simulink model "SwarmOptimizer"  (R2020a)
settings: Solver=VariableStepAuto  StartTime=0.0  StopTime=10.0  RelTol=1e-3
settings Model: Creator=PIM  LastModifiedBy=PIM

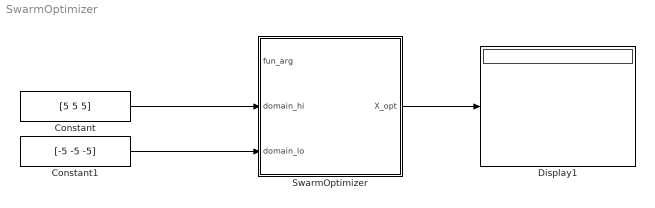
== system SwarmOptimizer ==
  Constant : Constant  Value=[5 5 5]  VectorParams1D=off
  Constant1 : Constant  Value=[-5 -5 -5]  VectorParams1D=off
  Display1 : Display
  SwarmOptimizer : Subsystem  mask{algorithm_mask=Differential Evolution Optimizer, n_iter=100, n_particles=50, sampling_method_mask=Uniform, dynamic_domain_flag=on, domain_hi_mask=[0 0 0], domain_lo_mask=[0 0 0]}
      mask prompts: algorithm_mask "Algorithm"; n_iter "Number of iterations [float]"; n_particles "Number of particles [float]"; sampling_method_mask "Sampling method"; dynamic_domain_flag "Dymamic Domain"; domain_hi_mask "Domain Hi (array) [float]"; domain_lo_mask "Domain Lo (array) [float]"
      mask init:
      | if strcmp(sampling_method_mask, 'Uniform')
      |     sampling_method=1;
      | elseif strcmp(sampling_method_mask, 'Cauchy')
      |     sampling_method=2;
      | elseif strcmp(sampling_method_mask, 'Normal')
      |     sampling_method=3;
      | end
      | 
      | if strcmp(algorithm_mask, 'Particle Swarm Optimizer')
      |     algorithm=1;
      | elseif strcmp(algorithm_mask, 'Differential Evolution Optimizer')
      |     algorithm=2;
      | end
      mask TypeOptions algorithm_mask: Particle Swarm Optimizer | Differential Evolution Optimizer
      mask TypeOptions sampling_method_mask: Uniform | Normal  | Cauchy
      mask DialogControl DescTextVar Prompt: Block to optimize a function using Swarm/Population based algorithms.
      mask DialogControl DescTextVar_copy Prompt: The function to be optimized is fun_opt(x, args)
      mask DialogControl DescTextVar_copy_copy Prompt: x: optimization variables (inputs)
      mask DialogControl DescTextVar_copy_copy_copy Prompt: args: disturbances
      mask DialogControl Control5 Prompt: Static Domain Definition
      mask Display: image('$imagefile'); % Use "Edit Image" on toolstrip to change.
  wires:
  SwarmOptimizer/1(X_opt) -> Display1/1
  Constant1/1 -> SwarmOptimizer/3(domain_lo)
  Constant/1 -> SwarmOptimizer/2(domain_hi)

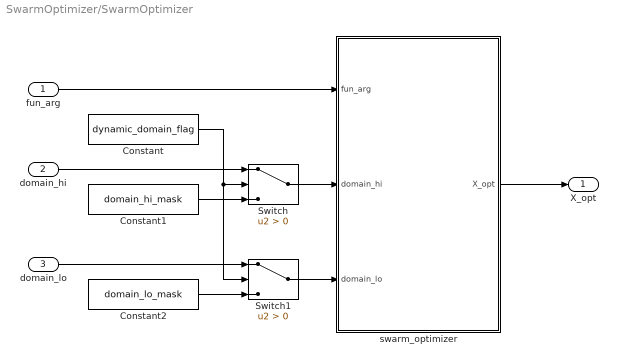
== system SwarmOptimizer/SwarmOptimizer ==
  fun_arg : Inport
  domain_hi : Inport  Port=2
  domain_lo : Inport  Port=3
  Constant : Constant  Value=dynamic_domain_flag
  Constant1 : Constant  Value=domain_hi_mask  VectorParams1D=off
  Constant2 : Constant  Value=domain_lo_mask  VectorParams1D=off
  Switch : Switch  Criteria=u2 > Threshold
  Switch1 : Switch  Criteria=u2 > Threshold
  swarm_optimizer : MATLAB Function  TreatAsAtomicUnit=on
  X_opt : Outport
  wires:
  domain_lo/1 -> Switch1/1
  Switch/1 -> swarm_optimizer/2(domain_hi)
  Constant2/1 -> Switch1/3
  Constant1/1 -> Switch/3
  Constant/1 -> Switch1/2, Switch/2
  domain_hi/1 -> Switch/1
  fun_arg/1 -> swarm_optimizer/1(fun_arg)
  Switch1/1 -> swarm_optimizer/3(domain_lo)
  swarm_optimizer/1(X_opt) -> X_opt/1

== matlab function SwarmOptimizer/swarm_optimizer ==
  data: fun_arg input; n_particles parameter int32; n_iter parameter int32; sampling_method parameter int8; algorithm parameter int8; X_opt output; domain_hi input double; domain_lo input double
function X_opt = swarm_optimizer(fun_arg, n_particles, n_iter, sampling_method, algorithm, domain_hi, domain_lo)
% global swarm_obj
% global topology_obj

swarm_obj=swarm;
topology_obj=topology;

%% Swarm parameters
swarm_param.n_particles=n_particles;
swarm_param.sampling_method='Uniform';
if sampling_method==1
    swarm_param.sampling_method='Uniform';
elseif sampling_method==2
    swarm_param.sampling_method='Cauchy';
elseif sampling_method==3
    swarm_param.sampling_method='Normal';
end
swarm_param.x_domain.hi=domain_hi;
swarm_param.x_domain.lo=domain_lo;

%% Algorithm parameters
alg_param.n_iter=n_iter;

alg_param.algorithm='ParticleSwarmOptimizer';
if algorithm==1
    alg_param.algorithm='ParticleSwarmOptimizer';
elseif algorithm==2
    alg_param.algorithm='DifferentialEvolutionOptimizer';
end


%% Specific configurations for Differential Evolution Algorithm
alg_param.CR    =0.9;       % crossover probability [0, 1]
alg_param.F     =0.8;       % differential weight [0, 2]

%% Specific configurations for Particle Swarm Optimizer Algorithm
alg_param.w     =0.1;       % velocity associated parameter
alg_param.c1    =0.1;       % personal best position coefficient
alg_param.c2    =0.2;       % global best position coefficient
alg_param.lr    =1;         % learning rate

X_opt=zeros(size(swarm_param.x_domain.hi));
if strcmp(alg_param.algorithm, 'DifferentialEvolutionOptimizer')
  [X_opt, y_opt]=DifferentialEvolutionOptimizer_codegen(alg_param, swarm_param, fun_arg);
end
  

end
